simulink model "dif_eq"  (R2020a)
settings: Solver=ode1  StartTime=0.0  StopTime=10.0  RelTol=1e-3
values from neighbouring files (symbols this model uses):
  omega_n = 2*pi/5    (= 1.25663706144)    [damping.m]    (also in damping_times_frequency.m = omega_ns(i); frequency.m = omega_ns(i); main.m; stepsize.m)
  xi = xis(i)    [damping.m]    (also in damping_times_frequency.m; frequency.m = 0.4; main.m = 0.4; stepsize.m = 0.4)
settings Model: Creator=josem  LastModifiedBy=josem

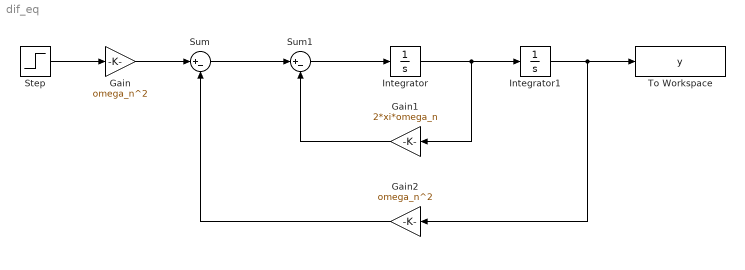
== system dif_eq ==
  Gain : Gain  Gain=omega_n^2
  Gain1 : Gain  Gain=2*xi*omega_n
  Gain2 : Gain  Gain=omega_n^2
  Integrator : Integrator
  Integrator1 : Integrator
  Step : Step  Time=0  SampleTime=0
  Sum : Sum  Inputs=|+-
  Sum1 : Sum  Inputs=|+-
  To Workspace : ToWorkspace  VariableName=y  SaveFormat=Structure With Time  SampleTime=-1
  wires:
  Step/1 -> Gain/1
  Gain/1 -> Sum/1
  Sum/1 -> Sum1/1
  Sum1/1 -> Integrator/1
  Integrator/1 -> Gain1/1, Integrator1/1
  Integrator1/1 -> Gain2/1, To Workspace/1
  Gain1/1 -> Sum1/2
  Gain2/1 -> Sum/2
